simulink model "Seguidor_discreto_plantilla"  (R2016a)
settings: Solver=VariableStepAuto  StartTime=0.0  StopTime=10  RelTol=1e-3
values from neighbouring files (symbols this model uses):
  Ki = K_dis(1:1,3:3)    [Regulador_seguidor_observador_codigo.m]
  Kp = K_dis(1:1,1:2)    [Regulador_seguidor_observador_codigo.m]
  tm = 0.1    [Regulador_seguidor_observador_codigo.m]
undefined symbols (not defined in the file or in its folder): A_dis, B_dis, C_dis
settings Model: Creator=Daniel  LastModifiedBy=Daniel

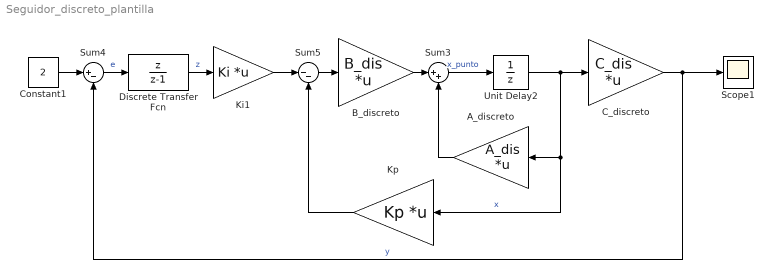
== system Seguidor_discreto_plantilla ==
  A_discreto : Gain  Gain=A_dis  Multiplication=Matrix(K*u) (u vector)
  B_discreto : Gain  Gain=B_dis  Multiplication=Matrix(K*u) (u vector)
  C_discreto : Gain  Gain=C_dis  Multiplication=Matrix(K*u) (u vector)
  Constant1 : Constant  Value=2
  Discrete Transfer Fcn : DiscreteTransferFcn  Numerator=[1 0]  Denominator=[1 -1]  SampleTime=tm
  Ki1 : Gain  Gain=Ki  Multiplication=Matrix(K*u) (u vector)
  Kp : Gain  Gain=Kp  Multiplication=Matrix(K*u) (u vector)
  Scope1 : Scope
  Sum3 : Sum  Inputs=|++
  Sum4 : Sum  Inputs=|+-
  Sum5 : Sum  Inputs=|--
  Unit Delay2 : UnitDelay  SampleTime=tm
  wires:
  Unit Delay2/1 -> Kp/1, A_discreto/1, C_discreto/1  "x"
  Sum3/1 -> Unit Delay2/1  "x_punto"
  A_discreto/1 -> Sum3/2
  Discrete Transfer Fcn/1 -> Ki1/1  "z"
  Sum4/1 -> Discrete Transfer Fcn/1  "e"
  C_discreto/1 -> Sum4/2, Scope1/1  "y"
  Constant1/1 -> Sum4/1
  Ki1/1 -> Sum5/1
  Sum5/1 -> B_discreto/1
  B_discreto/1 -> Sum3/1
  Kp/1 -> Sum5/2
